simulink model "cruise_control_sim"  (R2016b)
settings: Solver=ode1  StartTime=0.0  StopTime=50.0  FixedStep=0.1  RelTol=1e-3
PreLoadFcn:
  | load('cruise_control_sim.mat');
undefined symbols (not defined in the file): EngineRPM, EngineTRQ, FinalRatio, GearRatio, Kdrag, Ki, Kp, Mass, sigbuilder_block, WheelRadius
libraries: simulink x1
settings Model: Creator=bartb  LastModifiedBy=bartb

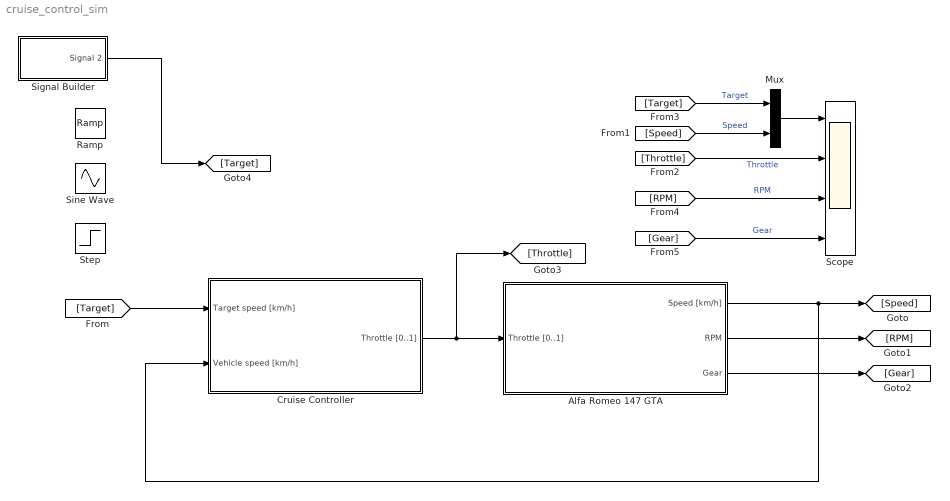
== system cruise_control_sim ==
  Alfa Romeo 147 GTA : Subsystem
  Cruise Controller : Subsystem
  Mux : Mux  Inputs=2
  Ramp : simulink/Sources/Ramp  slope=6  start=0  X0=0
  Scope : Scope  NumInputPorts=4
  Signal Builder : Subsystem  Tag=STV Subsys  LoadFcn=sigbuilder_block('load');  StartFcn=sigbuilder_block('start');  StopFcn=sigbuilder_block('stop');  ClipboardFcn=sigbuilder_block('clipboard');  mask(Sigbuilder block){tuvar=[0:10]}
      mask help: Simulink:masks:SigbuilderBlock_MD
      mask init:
      | if ~strcmp(get_param(bdroot(gcbh),'SimulationStatus'),'stopped') tuvar = sigbuilder_block('maskInit'); end
      settings: CopyFcn=sigbuilder_block('copy');  DeleteFcn=sigbuilder_block('delete');  ModelCloseFcn=sigbuilder_block('modelClose');  PreSaveFcn=sigbuilder_block('preSave');  PauseFcn=sigbuilder_block('pause');  ContinueFcn=sigbuilder_block('continue');  NameChangeFcn=sigbuilder_block('namechange');  OpenFcn=sigbuilder_block('open',[437.6 199.2 550.4 400 ]);  CloseFcn=sigbuilder_block('close');
      mask Display: plot(0, 0, 100, 100,[2, 2, 32, 32, 2], [68, 8, 8, 68, 68],[32, 2], [38, 38], [32, 19, 2],[53, 60, 44], [32, 17, 17, 2],[16, 16, 31, 31]);txt = getActiveGroup(gcbh);text(2, 100, txt,'verticalAlignment', 'top');
  Sine Wave : Sin  Amplitude=20  Bias=100  Frequency=0.2  SampleTime=0
  Step : Step  After=100  SampleTime=0
  wires:
  Cruise Controller/1(Throttle [0..1]) -> [Throttle], Alfa Romeo 147 GTA/1(Throttle [0..1])
  Alfa Romeo 147 GTA/1(Speed [km/h]) -> [Speed], Cruise Controller/2(Vehicle speed [km/h])
  Alfa Romeo 147 GTA/2(RPM) -> [RPM]
  Alfa Romeo 147 GTA/3(Gear) -> [Gear]
  [Target] -> Cruise Controller/1(Target speed [km/h])
  [Target] -> Mux/1  "Target"
  [Speed] -> Mux/2  "Speed"
  Mux/1 -> Scope/1
  [Throttle] -> Scope/2  "Throttle"
  [Gear] -> Scope/4  "Gear"
  [RPM] -> Scope/3  "RPM"
  Signal Builder/1(Signal 2) -> [Target]

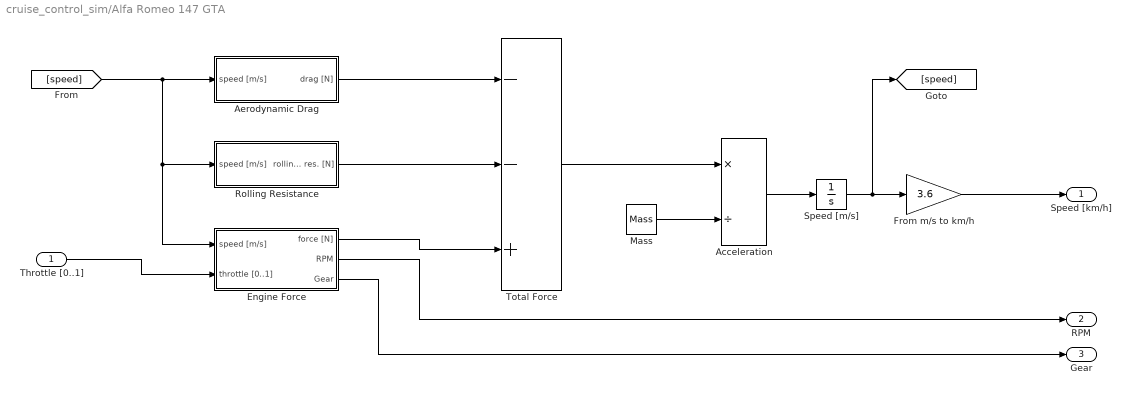
== system cruise_control_sim/Alfa Romeo 147 GTA ==
  Throttle [0..1] : Inport
  Acceleration : Product  Inputs=*/
  Aerodynamic Drag : Subsystem
  Engine Force : Subsystem
  From m/s to km/h : Gain  Gain=3.6
  Mass : Constant  Value=Mass
  Rolling Resistance : Subsystem
  Speed [m/s] : Integrator
  Total Force : Sum  Inputs=--+
  Speed [km/h] : Outport
  RPM : Outport  Port=2
  Gear : Outport  Port=3
  wires:
  Throttle [0..1]/1 -> Engine Force/2(throttle [0..1])
  Engine Force/1(force [N]) -> Total Force/3
  Rolling Resistance/1(rolling res. [N]) -> Total Force/2
  Aerodynamic Drag/1(drag [N]) -> Total Force/1
  Mass/1 -> Acceleration/2
  Total Force/1 -> Acceleration/1
  Acceleration/1 -> Speed [m/s]/1
  Speed [m/s]/1 -> [speed], From m/s to km/h/1
  From m/s to km/h/1 -> Speed [km/h]/1
  [speed] -> Engine Force/1(speed [m/s]), Rolling Resistance/1(speed [m/s]), Aerodynamic Drag/1(speed [m/s])
  Engine Force/2(RPM) -> RPM/1
  Engine Force/3(Gear) -> Gear/1

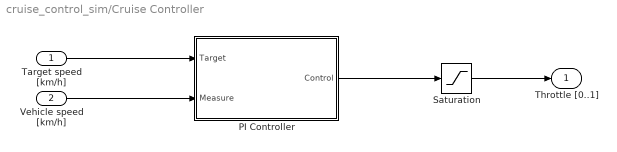
== system cruise_control_sim/Cruise Controller ==
  Target speed [km/h] : Inport
  Vehicle speed [km/h] : Inport  Port=2
  PI Controller : Subsystem
  Saturation : Saturate
  Throttle [0..1] : Outport
  wires:
  Saturation/1 -> Throttle [0..1]/1
  Vehicle speed [km/h]/1 -> PI Controller/2(Measure)
  Target speed [km/h]/1 -> PI Controller/1(Target)
  PI Controller/1(Control) -> Saturation/1

== system cruise_control_sim/Signal Builder ==
  Demux : Demux  Tag=STV Demux  Outputs=1
  FromWs : FromWorkspace  Tag=STV FromWs  VariableName=tuvar  SampleTime=0
      SigBuilderData=|
      | common.afterFinalStr = 'Extrapolate'
      | common.sampleTime = 0
      | dataSet.timeRange = [0 50]
      | dataSet.name = 'Group 1'
      | sbobj.Groups.Name = 'Group 1'
      | sbobj.Groups.Signals.Name = 'Signal 2'
      | sbobj.Groups.Signals.XData = [0 5 5 10 10 20 20 30 30 40 40 50]
      | sbobj.Groups.Signals.YData = [30 30 50 50 80 80 100 100 120 120 140 140]
      | sbobj.Groups.TimeRange = [0 50]
  Signal 2 : Outport  Tag=STV Outport
  wires:
  FromWs/1 -> Demux/1
  Demux/1 -> Signal 2/1

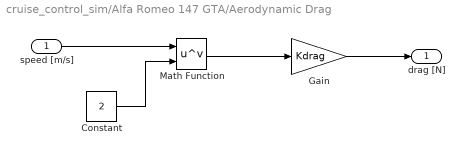
== system cruise_control_sim/Alfa Romeo 147 GTA/Aerodynamic Drag ==
  speed [m/s] : Inport
  Constant : Constant  Value=2
  Gain : Gain  Gain=Kdrag
  Math Function : Math  Operator=pow  SaturateOnIntegerOverflow=on
  drag [N] : Outport
  wires:
  speed [m/s]/1 -> Math Function/1
  Constant/1 -> Math Function/2
  Math Function/1 -> Gain/1
  Gain/1 -> drag [N]/1

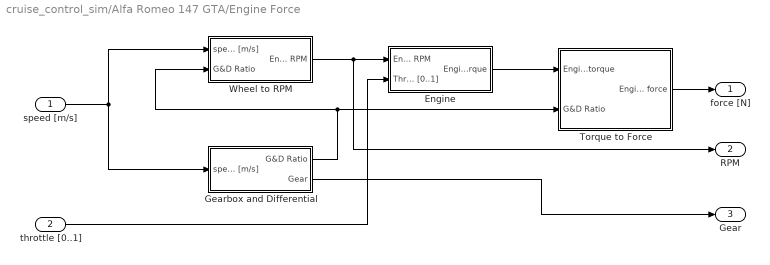
== system cruise_control_sim/Alfa Romeo 147 GTA/Engine Force ==
  speed [m/s] : Inport
  throttle [0..1] : Inport  Port=2
  Engine : Subsystem
  Gearbox and Differential : Subsystem
  Torque to Force : Subsystem
  Wheel to RPM : Subsystem
  force [N] : Outport
  RPM : Outport  Port=2
  Gear : Outport  Port=3
  wires:
  Wheel to RPM/1(Engine RPM) -> RPM/1, Engine/1(Engine RPM)
  speed [m/s]/1 -> Gearbox and Differential/1(speed [m/s]), Wheel to RPM/1(speed [m/s])
  Gearbox and Differential/1(G&D Ratio) -> Wheel to RPM/2(G&D Ratio), Torque to Force/2(G&D Ratio)
  throttle [0..1]/1 -> Engine/2(Throttle [0..1])
  Engine/1(Engine Torque) -> Torque to Force/1(Engine torque)
  Torque to Force/1(Engine force) -> force [N]/1
  Gearbox and Differential/2(Gear) -> Gear/1

== system cruise_control_sim/Alfa Romeo 147 GTA/Rolling Resistance ==
  speed [m/s] : Inport
  Gain : Gain  Gain=30 * Kdrag
  rolling res. [N] : Outport
  wires:
  speed [m/s]/1 -> Gain/1
  Gain/1 -> rolling res. [N]/1

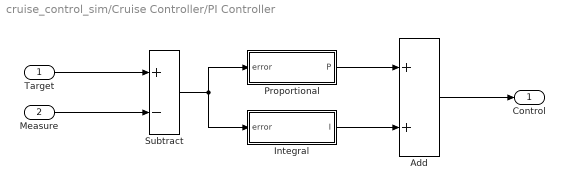
== system cruise_control_sim/Cruise Controller/PI Controller ==
  Target : Inport
  Measure : Inport  Port=2
  Add : Sum
  Integral : Subsystem
  Proportional : Subsystem
  Subtract : Sum  Inputs=+-
  Control : Outport
  wires:
  Subtract/1 -> Integral/1(error), Proportional/1(error)
  Integral/1(I) -> Add/2
  Measure/1 -> Subtract/2
  Add/1 -> Control/1
  Target/1 -> Subtract/1
  Proportional/1(P) -> Add/1

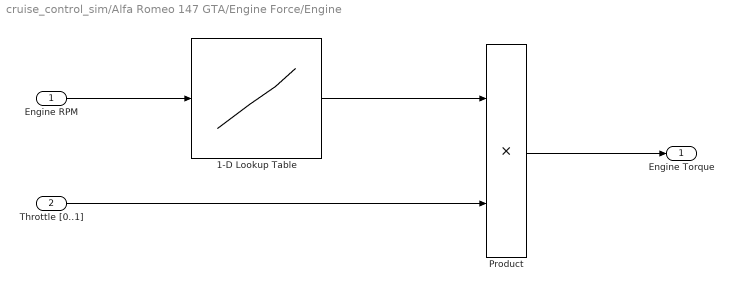
== system cruise_control_sim/Alfa Romeo 147 GTA/Engine Force/Engine ==
  Engine RPM : Inport
  Throttle [0..1] : Inport  Port=2
  1-D Lookup Table : Lookup_n-D  NumberOfTableDimensions=1  BreakpointsForDimension1=EngineRPM  Table=EngineTRQ  InterpMethod=Cubic spline  InternalRulePriority=Speed  RndMeth=Simplest  InputSameDT=on
  Product : Product
  Engine Torque : Outport
  wires:
  Engine RPM/1 -> 1-D Lookup Table/1
  1-D Lookup Table/1 -> Product/1
  Throttle [0..1]/1 -> Product/2
  Product/1 -> Engine Torque/1

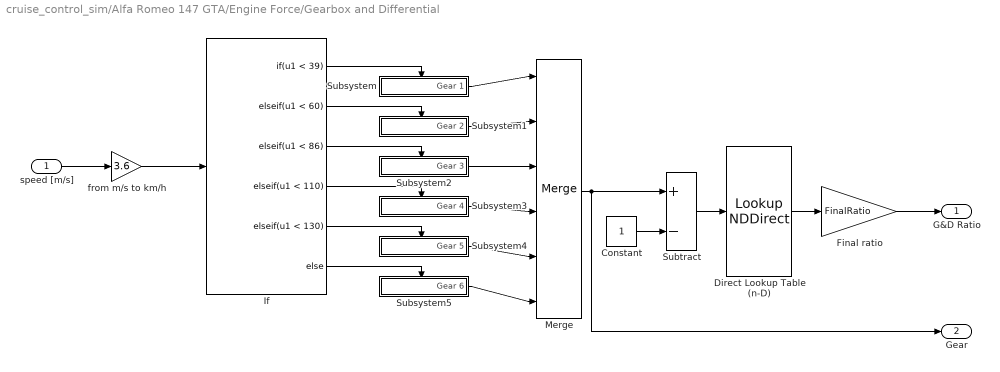
== system cruise_control_sim/Alfa Romeo 147 GTA/Engine Force/Gearbox and Differential ==
  speed [m/s] : Inport
  " Subsystem" : Subsystem  TreatAsAtomicUnit=on
  " Subsystem1" : Subsystem  TreatAsAtomicUnit=on
  " Subsystem2" : Subsystem  TreatAsAtomicUnit=on
  " Subsystem3" : Subsystem  TreatAsAtomicUnit=on
  " Subsystem4" : Subsystem  TreatAsAtomicUnit=on
  " Subsystem5" : Subsystem  TreatAsAtomicUnit=on
  Constant : Constant
  Direct Lookup Table (n-D) : LookupNDDirect  NumberOfTableDimensions=1  Table=GearRatio
  Final ratio : Gain  Gain=FinalRatio
  If : If  IfExpression=u1 < 39  ElseIfExpressions=u1 < 60, u1 < 86, u1 < 110, u1 < 130
  Merge : Merge  Inputs=6
  Subtract : Sum  Inputs=+-
  from m/s to km/h : Gain  Gain=3.6
  G&D Ratio : Outport
  Gear : Outport  Port=2
  wires:
  speed [m/s]/1 -> from m/s to km/h/1
  from m/s to km/h/1 -> If/1
  If/2 -> " Subsystem1"/Action
  If/3 -> " Subsystem2"/Action
  If/4 -> " Subsystem3"/Action
  If/5 -> " Subsystem4"/Action
  If/6 -> " Subsystem5"/Action
  If/1 -> " Subsystem"/Action
  " Subsystem"/1(Gear 1) -> Merge/1
  " Subsystem1"/1(Gear 2) -> Merge/2
  " Subsystem2"/1(Gear 3) -> Merge/3
  " Subsystem3"/1(Gear 4) -> Merge/4
  " Subsystem4"/1(Gear 5) -> Merge/5
  " Subsystem5"/1(Gear 6) -> Merge/6
  Constant/1 -> Subtract/2
  Merge/1 -> Gear/1, Subtract/1
  Subtract/1 -> Direct Lookup Table (n-D)/1
  Direct Lookup Table (n-D)/1 -> Final ratio/1
  Final ratio/1 -> G&D Ratio/1

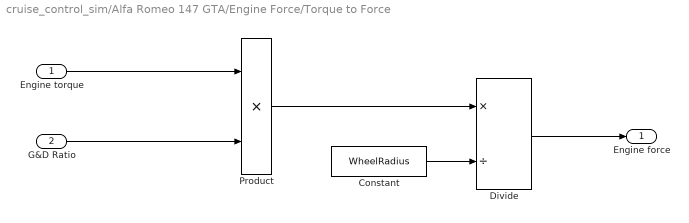
== system cruise_control_sim/Alfa Romeo 147 GTA/Engine Force/Torque to Force ==
  Engine torque : Inport
  G&D Ratio : Inport  Port=2
  Constant : Constant  Value=WheelRadius
  Divide : Product  Inputs=*/
  Product : Product
  Engine force : Outport
  wires:
  Engine torque/1 -> Product/1
  G&D Ratio/1 -> Product/2
  Constant/1 -> Divide/2
  Product/1 -> Divide/1
  Divide/1 -> Engine force/1

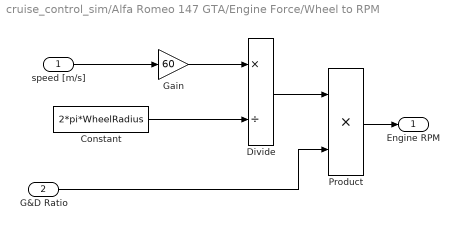
== system cruise_control_sim/Alfa Romeo 147 GTA/Engine Force/Wheel to RPM ==
  speed [m/s] : Inport
  G&D Ratio : Inport  Port=2
  Constant : Constant  Value=2*pi*WheelRadius
  Divide : Product  Inputs=*/
  Gain : Gain  Gain=60
  Product : Product
  Engine RPM : Outport
  wires:
  speed [m/s]/1 -> Gain/1
  Constant/1 -> Divide/2
  Gain/1 -> Divide/1
  Divide/1 -> Product/1
  G&D Ratio/1 -> Product/2
  Product/1 -> Engine RPM/1

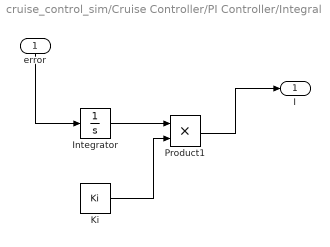
== system cruise_control_sim/Cruise Controller/PI Controller/Integral ==
  error : Inport
  Integrator : Integrator
  Ki : Constant  Value=Ki
  Product1 : Product
  I : Outport
  wires:
  Product1/1 -> I/1
  Integrator/1 -> Product1/1
  Ki/1 -> Product1/2
  error/1 -> Integrator/1

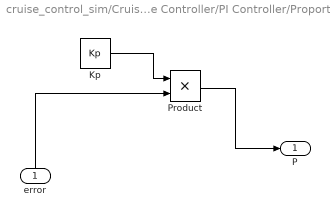
== system cruise_control_sim/Cruise Controller/PI Controller/Proportional ==
  error : Inport
  Kp : Constant  Value=Kp
  Product : Product
  P : Outport
  wires:
  Kp/1 -> Product/1
  Product/1 -> P/1
  error/1 -> Product/2

== system cruise_control_sim/Alfa Romeo 147 GTA/Engine Force/Gearbox and Differential/ Subsystem ==
  Action Port : ActionPort  ActionType=then
  Constant : Constant
  Gear 1 : Outport
  wires:
  Constant/1 -> Gear 1/1

== system cruise_control_sim/Alfa Romeo 147 GTA/Engine Force/Gearbox and Differential/ Subsystem1 ==
  Action Port : ActionPort  ActionType=elseif
  Constant : Constant  Value=2
  Gear 2 : Outport
  wires:
  Constant/1 -> Gear 2/1

== system cruise_control_sim/Alfa Romeo 147 GTA/Engine Force/Gearbox and Differential/ Subsystem2 ==
  Action Port : ActionPort  ActionType=elseif
  Constant : Constant  Value=3
  Gear 3 : Outport
  wires:
  Constant/1 -> Gear 3/1

== system cruise_control_sim/Alfa Romeo 147 GTA/Engine Force/Gearbox and Differential/ Subsystem3 ==
  Action Port : ActionPort  ActionType=elseif
  Constant : Constant  Value=4
  Gear 4 : Outport
  wires:
  Constant/1 -> Gear 4/1

== system cruise_control_sim/Alfa Romeo 147 GTA/Engine Force/Gearbox and Differential/ Subsystem4 ==
  Action Port : ActionPort  ActionType=elseif
  Constant : Constant  Value=5
  Gear 5 : Outport
  wires:
  Constant/1 -> Gear 5/1

== system cruise_control_sim/Alfa Romeo 147 GTA/Engine Force/Gearbox and Differential/ Subsystem5 ==
  Action Port : ActionPort  ActionType=else
  Constant : Constant  Value=6
  Gear 6 : Outport
  wires:
  Constant/1 -> Gear 6/1
